simulink model "switch_operations"  (R2024b)
settings: Solver=ode3  StartTime=0.0  StopTime=10.0  FixedStep=0.01  RelTol=1e-3
settings Model: Creator=balaj  LastModifiedBy=balaj

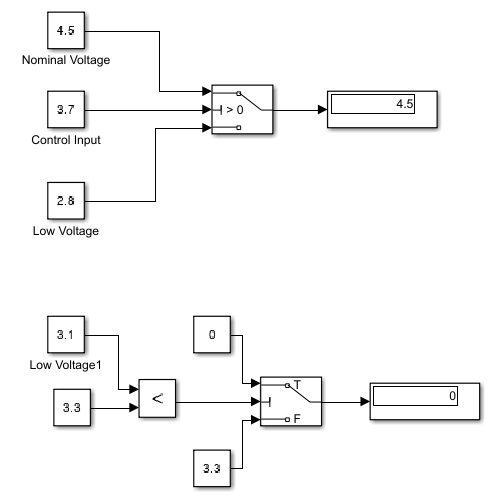
[thumbnail: Simulink's stored preview of the top-level diagram]
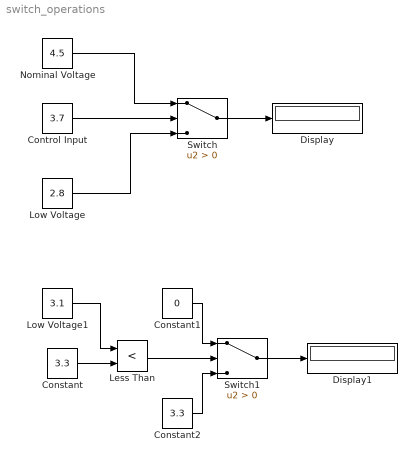
== system switch_operations ==
  Constant : Constant  Value=3.3
  Constant1 : Constant  Value=0
  Constant2 : Constant  Value=3.3
  Control Input : Constant  Value=3.7  SampleTime=1
  Display : Display
  Display1 : Display
  Less Than : RelationalOperator  Operator=<  OutDataTypeStr=boolean  RndMeth=Simplest  InputSameDT=off
  Low Voltage : Constant  Value=2.8  SampleTime=1
  Low Voltage1 : Constant  Value=3.1  SampleTime=1
  Nominal Voltage : Constant  Value=4.5  SampleTime=1
  Switch : Switch  Criteria=u2 > Threshold  SaturateOnIntegerOverflow=off  InputSameDT=off
  Switch1 : Switch  Criteria=u2 > Threshold  SaturateOnIntegerOverflow=off  InputSameDT=off
  wires:
  Control Input/1 -> Switch/2
  Nominal Voltage/1 -> Switch/1
  Low Voltage/1 -> Switch/3
  Switch/1 -> Display/1
  Low Voltage1/1 -> Less Than/1
  Constant/1 -> Less Than/2
  Less Than/1 -> Switch1/2
  Constant1/1 -> Switch1/1
  Constant2/1 -> Switch1/3
  Switch1/1 -> Display1/1
